simulink model "GEN__S3_2_PI"  (R2024a)
settings: Solver=VariableStepAuto  StartTime=0.0  StopTime=10.0  RelTol=1e-3
settings Model: Creator=edub  LastModifiedBy=edub

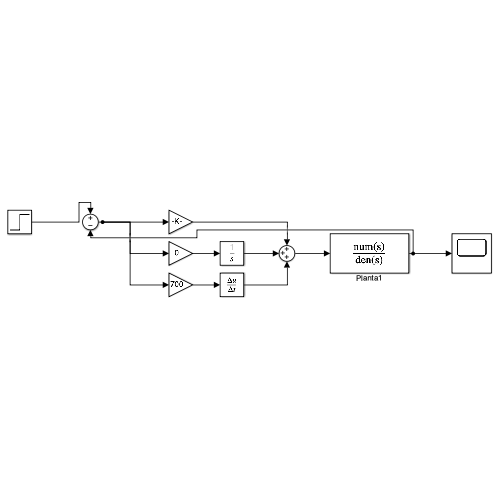
[thumbnail: Simulink's stored preview of the top-level diagram]
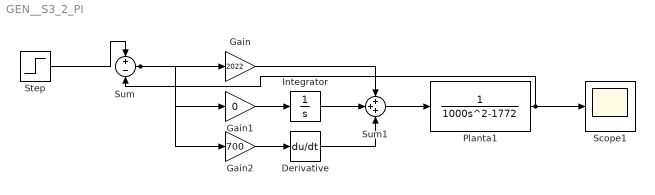
== system GEN__S3_2_PI ==
  Derivative : Derivative
  Gain : Gain  Gain=2022
  Gain1 : Gain  Gain=0
  Gain2 : Gain  Gain=700
  Integrator : Integrator
  Planta1 : TransferFcn  Numerator=[0 0 1]  Denominator=[1000 0 -1772]
  Scope1 : Scope
  Step : Step  SampleTime=0
  Sum : Sum  Inputs=+-
  Sum1 : Sum  Inputs=+++
  wires:
  Step/1 -> Sum/1
  Sum/1 -> Gain/1, Gain1/1, Gain2/1
  Gain/1 -> Sum1/1
  Gain1/1 -> Integrator/1
  Integrator/1 -> Sum1/2
  Gain2/1 -> Derivative/1
  Derivative/1 -> Sum1/3
  Sum1/1 -> Planta1/1
  Planta1/1 -> Scope1/1, Sum/2
